simulink model "three_phase_inverter_with_spwm"  (R2024b)
settings: Solver=ode3  StartTime=0.0  StopTime=0.10  FixedStep=10e-6  RelTol=1e-3
libraries: spsIGBTLib x6, spsVoltageMeasurementLib x3, spsDCVoltageSourceLib x1, spsGroundLib x1, spsThreePhaseParallelRLCBranchLib x1, spsThreePhaseVIMeasurementLib x1, spsTriangleGeneratorLib x1, sps_lib x1
settings Model: Creator=PRASHANTH  LastModifiedBy=Abhijith_Kumble

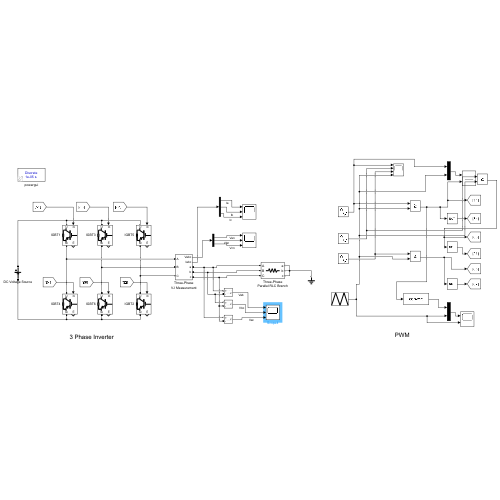
[thumbnail: Simulink's stored preview of the top-level diagram]
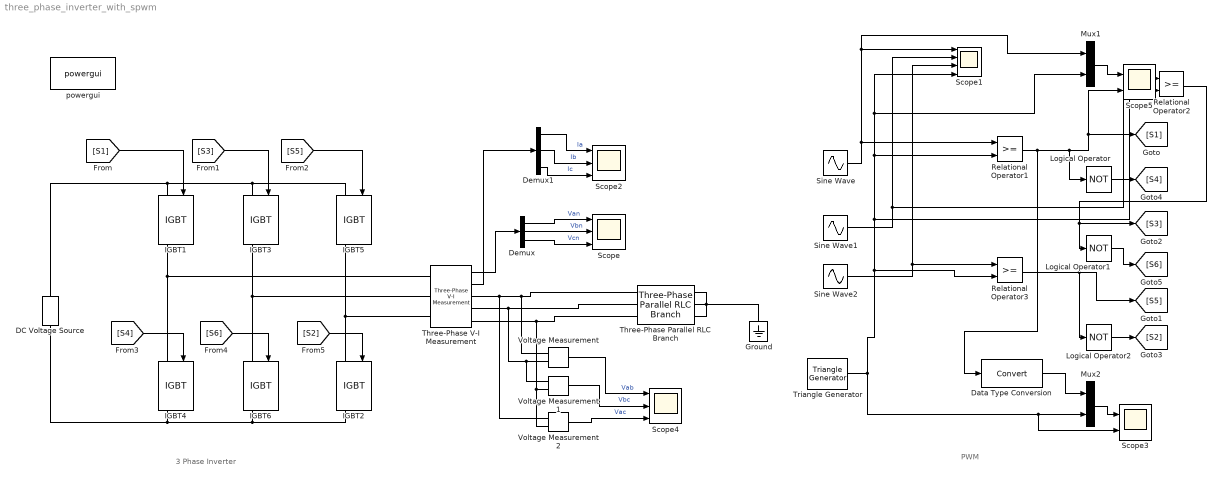
== system three_phase_inverter_with_spwm ==
  note: PWM
  note: 3 Phase Inverter
  DC Voltage Source : spsDCVoltageSourceLib/DC Voltage Source  Amplitude=415  Measurements=None
  Data Type Conversion : DataTypeConversion  SaturateOnIntegerOverflow=off  RndMeth=Floor
  Demux : Demux  Outputs=3
  Demux1 : Demux  Outputs=3
  Ground : spsGroundLib/Ground  LConnTagsString=a
  IGBT{1..6} (6 alike) : spsIGBTLib/IGBT  Ron=0.001  Lon=0  Vf=1  Tf=1e-6  Tt=2e-6  IC=0  Rs=1e5  Cs=inf  Measurements=on
  Logical Operator : Logic  Operator=NOT  AllPortsSameDT=off  OutDataTypeStr=boolean
  Logical Operator1 : Logic  Operator=NOT  AllPortsSameDT=off  OutDataTypeStr=boolean
  Logical Operator2 : Logic  Operator=NOT  AllPortsSameDT=off  OutDataTypeStr=boolean
  Mux1 : Mux  Inputs=2
  Mux2 : Mux  Inputs=2
  Relational Operator1 : RelationalOperator  OutDataTypeStr=boolean  InputSameDT=off
  Relational Operator2 : RelationalOperator  OutDataTypeStr=boolean  InputSameDT=off
  Relational Operator3 : RelationalOperator  OutDataTypeStr=boolean  InputSameDT=off
  Scope : Scope  NumInputPorts=3
  Scope1 : Scope  NumInputPorts=4
  Scope2 : Scope  NumInputPorts=3
  Scope3 : Scope  NumInputPorts=2
  Scope4 : Scope  NumInputPorts=3
  Scope5 : Scope  NumInputPorts=2
  Sine Wave : Sin  Frequency=2*pi*50  SampleTime=0
  Sine Wave1 : Sin  Frequency=2*pi*50  Phase=2*pi/3  SampleTime=0
  Sine Wave2 : Sin  Frequency=2*pi*50  Phase=-2*pi/3  SampleTime=0
  Three-Phase Parallel RLC Branch : spsThreePhaseParallelRLCBranchLib/Three-Phase Parallel RLC Branch  LConnTagsString=A|B|C  RConnTagsString=A|B|C  BranchType=R  Resistance=1e3  Inductance=1e-3  Capacitance=1e-6  Measurements=None
  Three-Phase V-I Measurement : spsThreePhaseVIMeasurementLib/Three-Phase V-I Measurement  VoltageMeasurement=phase-to-ground  SetLabelV=off  LabelV=Vabc  Vpu=off  VpuLL=off  CurrentMeasurement=yes  SetLabelI=off  LabelI=Iabc  Ipu=off  Pbase=100e6  Vbase=500e3  OutputType=Complex  PhasorSimulation=off  PSBequivalent=0
  Triangle Generator : spsTriangleGeneratorLib/Triangle Generator  Freq=1e3  Phase=0  Ts=0
  Voltage Measurement : spsVoltageMeasurementLib/Voltage Measurement  PhasorSimulation=off  OutputType=Complex  PSBequivalent=0
  Voltage Measurement1 : spsVoltageMeasurementLib/Voltage Measurement  PhasorSimulation=off  OutputType=Complex  PSBequivalent=0
  Voltage Measurement2 : spsVoltageMeasurementLib/Voltage Measurement  PhasorSimulation=off  OutputType=Complex  PSBequivalent=0
  powergui : sps_lib/powergui  Priority=1  SimulationMode=Discrete  SampleTime=10e-6  frequency=60  Iterations=50  frequencyindice=0  Pbase=100e6  ErrMax=1e-4  UnitsV=kV  UnitsW=MW  buscounter=0  FunctionMessages=off  echomessages=off  EnableUseOfTLC=off  CurrentSourceSwitches=off  DisableSnubberDevices=off  DisableRonSwitches=off  DisableVfSwitches=off  DisplayEquations=off  AutomaticDiscreteSolvers=off  SolverType=Tustin/Backward Euler (TBE)  Interpol=off  ExternalGateDelay=off  methode=off  Ts=100  x0status=blocks  SPID=on  SwTol=0  HookPort=off  NonlinearTolerance=1e-4  nMaxIteration=100  ContinueOnMaxIteration=off  RestoreLinks=warning  ResistiveCurrentMeasurement=off  Frange=[0:2:500]  Ylog=off  Xlog=on  ShowGrid=off  save=off  variable=ZData  structure=0  ZoomFFT=off  StartTime=0.0  cycles=1  DisplayStyle=1  fundamental=60  FreqAxis=off  MaxFrequency=1000  frequencyindicesteady=1  RmsSteady=1  display=off
  wires:
  [S1] -> IGBT1/1
  [S3] -> IGBT3/1
  [S5] -> IGBT5/1
  [S4] -> IGBT4/1
  [S6] -> IGBT6/1
  [S2] -> IGBT2/1
  Three-Phase V-I Measurement/1 -> Demux/1
  Demux/1 -> Scope/1  "Van"
  Demux/2 -> Scope/2  "Vbn"
  Demux/3 -> Scope/3  "Vcn"
  Triangle Generator/1 -> Scope3/2, Mux2/2, Scope1/4, Mux1/2, Relational Operator1/2, Relational Operator2/2, Relational Operator3/2
  Mux2/1 -> Scope3/1
  Sine Wave2/1 -> Scope1/3, Relational Operator3/1
  Logical Operator/1 -> [S4]
  Data Type Conversion/1 -> Mux2/1
  Sine Wave/1 -> Scope1/1, Mux1/1, Relational Operator1/1
  Relational Operator1/1 -> Data Type Conversion/1, Scope5/2, [S1], Logical Operator/1
  Sine Wave1/1 -> Scope1/2, Relational Operator2/1
  Mux1/1 -> Scope5/1
  Relational Operator2/1 -> [S3], Logical Operator1/1
  Relational Operator3/1 -> [S5], Logical Operator2/1
  Logical Operator1/1 -> [S6]
  Logical Operator2/1 -> [S2]
  Three-Phase V-I Measurement/2 -> Demux1/1
  Demux1/1 -> Scope2/1  "Ia"
  Demux1/2 -> Scope2/2  "Ib"
  Demux1/3 -> Scope2/3  "Ic"
  Voltage Measurement/1 -> Scope4/1  "Vab"
  Voltage Measurement2/1 -> Scope4/3  "Vac"
  Voltage Measurement1/1 -> Scope4/2  "Vbc"
  connections:
  DC Voltage Source/RConn1 -- IGBT5/LConn1 -- IGBT3/LConn1 -- IGBT1/LConn1
  DC Voltage Source/LConn1 -- IGBT2/RConn1 -- IGBT6/RConn1 -- IGBT4/RConn1
  IGBT1/RConn1 -- Three-Phase V-I Measurement/LConn1 -- IGBT4/LConn1
  IGBT3/RConn1 -- Three-Phase V-I Measurement/LConn2 -- IGBT6/LConn1
  IGBT5/RConn1 -- Three-Phase V-I Measurement/LConn3 -- IGBT2/LConn1
  Three-Phase V-I Measurement/RConn1 -- Voltage Measurement2/LConn1 -- Voltage Measurement/LConn1 -- Three-Phase Parallel RLC Branch/LConn1
  Three-Phase Parallel RLC Branch/LConn2 -- Voltage Measurement1/LConn1 -- Voltage Measurement/LConn2 -- Three-Phase V-I Measurement/RConn2
  Three-Phase Parallel RLC Branch/LConn3 -- Voltage Measurement2/LConn2 -- Voltage Measurement1/LConn2 -- Three-Phase V-I Measurement/RConn3
  Three-Phase Parallel RLC Branch/RConn1 -- Ground/LConn1 -- Three-Phase Parallel RLC Branch/RConn2 -- Three-Phase Parallel RLC Branch/RConn3
